simulink library "RelHum2x"  (R2018b)
settings: Solver=ode45  StartTime=0.0  StopTime=10.0  RelTol=1e-3  EnableMultiTasking=on
libraries: carnot x1
settings Model: Creator=lena.frank  LastModifiedBy=drhf
settings DataIOCC: LimitDataPoints=on  SaveFormat=Array  SignalLoggingSaveFormat=ModelDataLogs
settings OptimizationCC: ExpressionDepthLimit=2147483647  LifeSpan=inf
settings DebuggingCC: UnderspecifiedInitializationDetection=Classic  MergeDetectMultiDrivingBlocksExec=none  SolverPrmCheckMsg=warning  FcnCallInpInsideContextMsg=warning  StateNameClashWarn=warning  SFUnexpectedBacktrackingDiag=warning  SFNoUnconditionalDefaultTransitionDiag=warning  SFExecutionAtInitializationDiag=none
settings HardwareCC: ProdBitPerPointer=32  ProdBitPerSizeT=32  ProdBitPerPtrDiffT=32  ProdLargestAtomicFloat=None  ProdIntDivRoundTo=Undefined  ProdEndianess=Unspecified  ProdWordSize=32  ProdHWDeviceType=32-bit Generic
settings ModelReferenceCC: PropagateSignalLabelsOutOfModel=off
settings SFSimCC: SimUseLocalCustomCode=off
settings RTWCC: RTWUseLocalCustomCode=off
settings CodeAppCC: StateflowObjectComments=on
settings GRTTargetCC: TargetLangStandard=C89/C90 (ANSI)  GeneratePreprocessorConditionals=Disable all  CombineOutputUpdateFcns=off  GRTInterface=on
settings ConfigComp: CovMetricSettings=dw  CovHtmlReporting=on  CovSaveCumulativeToWorkspaceVar=on  CovSaveSingleToWorkspaceVar=on  CovExternalEMLEnable=off

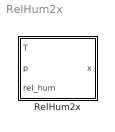
== system RelHum2x ==
  RelHum2x : Subsystem  mask(relative humidity to x){}
      mask help:
      | Calculate the mass of water per mass of air (x)
      | from the relative humidity of air.
      |
      | T             [degree centigrade]
      | p             [Pa]
      | rel_hum   [percent]
      | x              kg water / kg air
      mask Help: web(fullfile(path_carnot('help'),'RelHum2x.html'),'-helpbrowser')

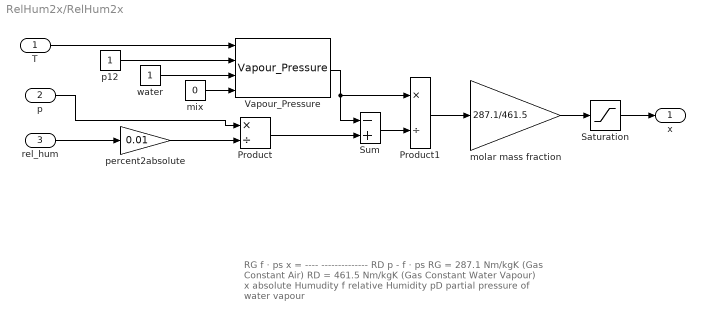
== system RelHum2x/RelHum2x ==
  note: RG      f · ps
      |  x  = ----  --------------
      |         RD     p - f · ps
      |
      | RG = 287.1 Nm/kgK (Gas Constant Air)
      | RD = 461.5 Nm/kgK (Gas Constant Water Vapour)
      | x absolute Humudity
      | f relative Humidity
      | pD partial pressure of water vapour
  T : Inport
  p : Inport  Port=2
  rel_hum : Inport  Port=3
  Product : Product  Inputs=*/  SaturateOnIntegerOverflow=on  InputSameDT=on  OutDataTypeStr=Inherit: Same as first input
  Product1 : Product  Inputs=*/  SaturateOnIntegerOverflow=on  InputSameDT=on  OutDataTypeStr=Inherit: Same as first input
  Saturation : Saturate  UpperLimit=inf  LowerLimit=0
  Sum : Sum  Inputs=-+  SaturateOnIntegerOverflow=on  InputSameDT=on  OutDataTypeStr=Inherit: Same as first input
  Vapour_Pressure : carnot/Basic/Material_Properties/Vapour_Pressure  VariantControl=CarlibClassic  INPUTARGUMENTS=state variables (classic)  DEBUGLEVEL=WARNINGLEVEL  MAXTOTALMESSAGES=inf  MAXCONSECUTIVEMESSAGES=inf  WRITETOFILE=0  FILENAME='errors.txt'
      settings: SourceProductName=Carnot
  mix : Constant  Value=0
  molar mass fraction : Gain  Gain=287.1/461.5  SaturateOnIntegerOverflow=on  OutDataTypeStr=Inherit: Same as input  ParamDataTypeStr=Inherit: Same as input
  p12 : Constant
  percent2absolute : Gain  Gain=0.01  SaturateOnIntegerOverflow=on  OutDataTypeStr=Inherit: Same as input  ParamDataTypeStr=Inherit: Same as input
  water : Constant
  x : Outport
  wires:
  Saturation/1 -> x/1
  molar mass fraction/1 -> Saturation/1
  percent2absolute/1 -> Product/2
  rel_hum/1 -> percent2absolute/1
  Vapour_Pressure/1 -> Product1/1, Sum/1
  mix/1 -> Vapour_Pressure/4
  p12/1 -> Vapour_Pressure/2
  water/1 -> Vapour_Pressure/3
  T/1 -> Vapour_Pressure/1
  Product1/1 -> molar mass fraction/1
  Sum/1 -> Product1/2
  Product/1 -> Sum/2
  p/1 -> Product/1
